simulink model "IMSPM_Q36121333_LAB3_SYSTEM"  (R2021b)
settings: Solver=ode45  StartTime=0.0  StopTime=0.015  MaxStep=1e-8  RelTol=1e-3
undefined symbols (not defined in the file): plecs
libraries: modelsimlib x1
settings Model: Creator=stanl  LastModifiedBy=stanl

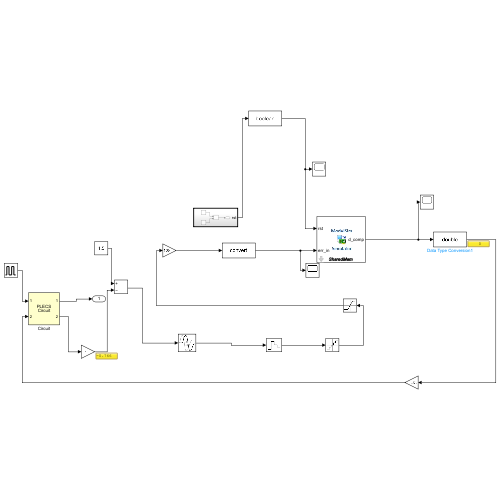
[thumbnail: Simulink's stored preview of the top-level diagram]
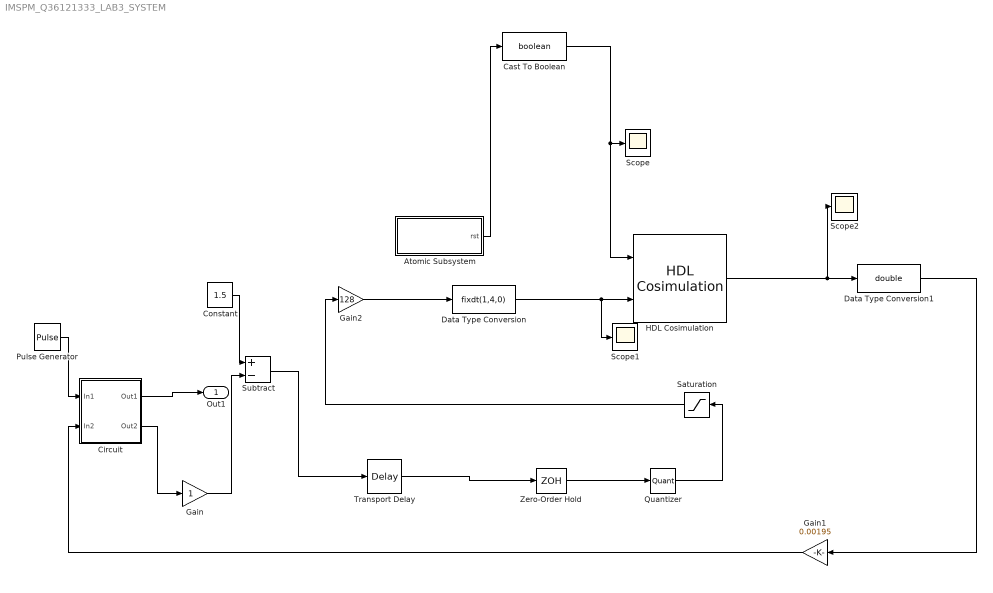
== system IMSPM_Q36121333_LAB3_SYSTEM ==
  Atomic Subsystem : Subsystem  TreatAsAtomicUnit=on
  Cast To Boolean : DataTypeConversion  OutDataTypeStr=boolean
  Circuit : Subsystem  LoadFcn=plecs('sl', 200);  InitFcn=plecs('sl', 214);  StartFcn=plecs('sl', 208);  StopFcn=plecs('sl', 209);  mask(PlecsCircuit){PLECSData=<binary blob, 3624 chars, not shown>}
      mask prompts: PLECSData "PLECS Data (Do not delete or modify!)"
      mask init:
      | % PLACE CUSTOM INITIALIZATIONS ABOVE
      | % DO NOT REMOVE
      | plecs('sl', 215);
      | % DO NOT REMOVE
      settings: CopyFcn=plecs('sl', 203);  DeleteFcn=plecs('sl', 205);  UndoDeleteFcn=plecs('sl', 206);  PreSaveFcn=plecs('sl', 211);  PostSaveFcn=plecs('sl', 201);  NameChangeFcn=plecs('sl', 210);  DestroyFcn=plecs('sl', 207);  PreCopyFcn=plecs('sl', 216);  OpenFcn=plecs('sl', 202);  ErrorFcn=plerrorfcn
      mask Help: web(['file:///' fullfile(plecsdoc, 'creatingacircuit.html')])
      mask Display: disp('PLECS\nCircuit')
  Constant : Constant  Value=1.5
  Data Type Conversion : DataTypeConversion  OutDataTypeStr=fixdt(1,4,0)
  Data Type Conversion1 : DataTypeConversion  OutDataTypeStr=double
  Gain : Gain
  Gain1 : Gain  Gain=0.00195
  Gain2 : Gain  Gain=128
  HDL Cosimulation : modelsimlib/HDL Cosimulation  PortPaths=/compensator/rst;/compensator/err_in;/compensator/d_comp  PortModes=[1 1 2 ]  PortTimes=[-1,-1,2e-6]  PortSigns=[-1 -1 -1 ]  PortFracLengths=[0,0,0]  CommLocal=on  CommSharedMemory=on  CommPortNumber=4449  CommShowInfo=on  ClockPaths=/compensator/clk  ClockModes=[2 ]  ClockTimes=[1e-6]  TclPreSimCommand="puts \"Running Simulink Cosimulation block.\""  TclPostSimCommand="puts \"done\""  TimingMode=s  TimingScaleFactor=1  idxCellArray={'UNUSED_VAR'}  CosimBypass=Full Simulation  AllowDirectFeedthrough=on  ProductName=EDA Simulator Link MQ  RunAutoTimescale=off  HdlClocks=0  PreRunTime=0  PreRunTimeUnit=ns
      settings: SourceProductBaseCode=ES
  Pulse Generator : DiscretePulseGenerator  PulseType=Time based  Amplitude=5  Period=0.002  PulseWidth=50  PhaseDelay=0.0005
  Quantizer : Quantizer  QuantizationInterval=0.0078125
  Saturation : Saturate  UpperLimit=0.03125  LowerLimit=-0.03125
  Scope : Scope
  Scope1 : Scope
  Scope2 : Scope
  Subtract : Sum  Inputs=+-
  Transport Delay : TransportDelay  DelayTime=7e-7  InitialOutput=1.5  PadeOrder=2
  Zero-Order Hold : ZeroOrderHold  SampleTime=2e-6
  Out1 : Outport
  wires:
  HDL Cosimulation/1 -> Scope2/1, Data Type Conversion1/1
  Subtract/1 -> Transport Delay/1
  Transport Delay/1 -> Zero-Order Hold/1
  Circuit/2(Out2) -> Gain/1
  Gain2/1 -> Data Type Conversion/1
  Atomic Subsystem/1(rst) -> Cast To Boolean/1
  Saturation/1 -> Gain2/1
  Constant/1 -> Subtract/1
  Pulse Generator/1 -> Circuit/1(In1)
  Gain1/1 -> Circuit/2(In2)
  Circuit/1(Out1) -> Out1/1
  Gain/1 -> Subtract/2
  Quantizer/1 -> Saturation/1
  Data Type Conversion1/1 -> Gain1/1
  Zero-Order Hold/1 -> Quantizer/1
  Cast To Boolean/1 -> HDL Cosimulation/1, Scope/1
  Data Type Conversion/1 -> Scope1/1, HDL Cosimulation/2

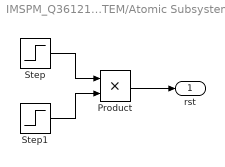
== system IMSPM_Q36121333_LAB3_SYSTEM/Atomic Subsystem ==
  Product : Product
  Step : Step  Time=0.5e-6  SampleTime=1e-8
  Step1 : Step  Time=0.8e-6  Before=1  After=0  SampleTime=1e-8
  rst : Outport
  wires:
  Step1/1 -> Product/2
  Step/1 -> Product/1
  Product/1 -> rst/1

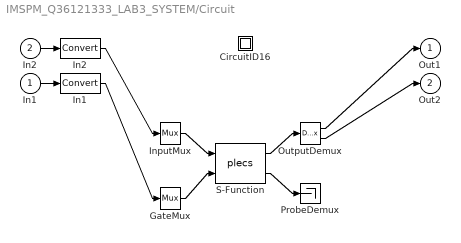
== system IMSPM_Q36121333_LAB3_SYSTEM/Circuit ==
  In1 : Inport  PortDimensions=1
  In2 : Inport  Port=2  PortDimensions=1
  " CircuitID16 " : Subsystem
  " GateMux " : Mux  Inputs=[ 1 ]
  " In1 " : DataTypeConversion  SaturateOnIntegerOverflow=on  RndMeth=Zero
  " In2 " : DataTypeConversion  SaturateOnIntegerOverflow=on  RndMeth=Zero
  " InputMux " : Mux  Inputs=[ 1 ]
  " OutputDemux " : Demux  Outputs=[ 1 1 ]
  " ProbeDemux " : Terminator
  " S-Function " : S-Function  FunctionName=plecs  SFunctionDeploymentMode=off  EnableBusSupport=off
  Out1 : Outport  PortDimensions=1
  Out2 : Outport  Port=2  PortDimensions=1
  wires:
  " InputMux "/1 -> " S-Function "/1
  " GateMux "/1 -> " S-Function "/2
  " S-Function "/1 -> " OutputDemux "/1
  " S-Function "/2 -> " ProbeDemux "/1
  In2/1 -> " In2 "/1
  " In2 "/1 -> " InputMux "/1
  In1/1 -> " In1 "/1
  " In1 "/1 -> " GateMux "/1
  " OutputDemux "/1 -> Out1/1
  " OutputDemux "/2 -> Out2/1

== system IMSPM_Q36121333_LAB3_SYSTEM/Circuit/ CircuitID16  ==
